simulink model "PV_MG_DroopMPPTV3_TwoFarms_VariableDT_VariableSampling"  (R2015a)
settings: Solver=ode3  StartTime=0.0  StopTime=inf  FixedStep=DT  RelTol=1e-3
undefined symbols (not defined in the file): CT, DT, Ion, Lithium
libraries: powerlib x61, powerlib_meascontrol x12, simulink x10, fuzblock x3, simulink_extras x3, re_lib x2, electricdrivelib x1
(part 2 of 2)

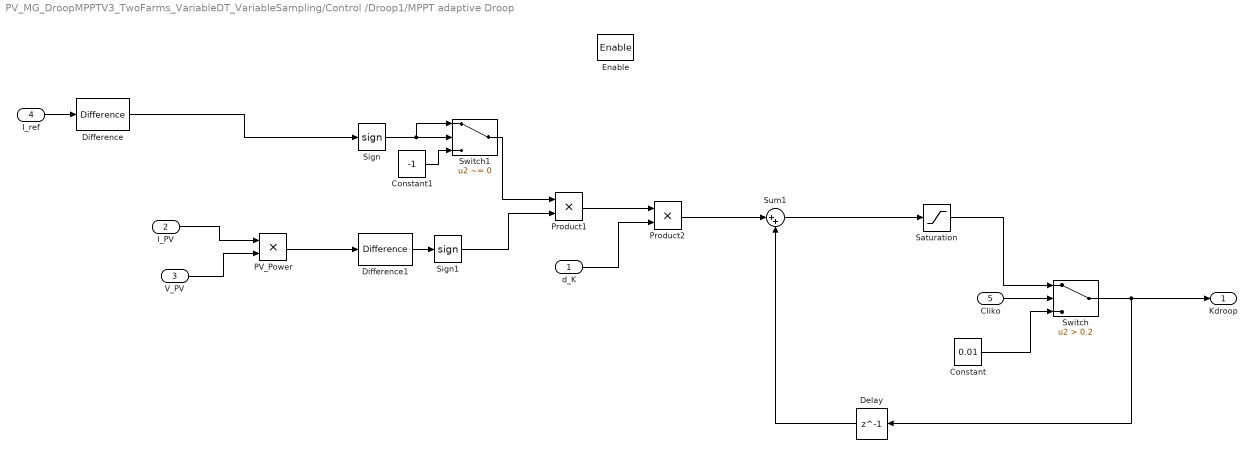
== system PV_MG_DroopMPPTV3_TwoFarms_VariableDT_VariableSampling/Control /Droop1/MPPT adaptive Droop ==
  d_K : Inport  SampleTime=CT
  I_PV : Inport  Port=2  SampleTime=CT
  V_PV : Inport  Port=3  SampleTime=CT
  I_ref : Inport  Port=4  SampleTime=CT
  "Cliko " : Inport  Port=5  SampleTime=CT
  Enable : EnablePort
  Constant : Constant  Value=0.01  SampleTime=CT
  Constant1 : Constant  Value=-1  SampleTime=CT
  Delay : Delay  DelayLength=1  InitialCondition=0  SampleTime=CT
  Difference : simulink/Discrete/Difference  ICPrevInput=0.0  InputProcessing=Inherited  OutMin=[]  OutMax=[]  OutDataType=fixdt(1, 16)  OutScaling=2^-10  DoSatur=off
  Difference1 : simulink/Discrete/Difference  ICPrevInput=0.0  InputProcessing=Inherited  OutMin=[]  OutMax=[]  OutDataType=fixdt(1, 16)  OutScaling=2^-10  DoSatur=off
  PV_Power : Product
  Product1 : Product
  Product2 : Product
  Saturation : Saturate  UpperLimit=4  LowerLimit=0
  Sign : Signum
  Sign1 : Signum
  Sum1 : Sum  Inputs=|++
  Switch : Switch  Criteria=u2 > Threshold  Threshold=0.2
  Switch1 : Switch  Criteria=u2 ~= 0  Threshold=0.1
  Kdroop : Outport  SampleTime=CT
  wires:
  I_ref/1 -> Difference/1
  V_PV/1 -> PV_Power/2
  I_PV/1 -> PV_Power/1
  Difference/1 -> Sign/1
  Switch1/1 -> Product1/1
  Constant1/1 -> Switch1/3
  Sign/1 -> Switch1/2, Switch1/1
  Saturation/1 -> Switch/1
  Constant/1 -> Switch/3
  Sum1/1 -> Saturation/1
  Delay/1 -> Sum1/2
  Product2/1 -> Sum1/1
  d_K/1 -> Product2/2
  Product1/1 -> Product2/1
  Sign1/1 -> Product1/2
  Difference1/1 -> Sign1/1
  PV_Power/1 -> Difference1/1
  Switch/1 -> Delay/1, Kdroop/1
  "Cliko "/1 -> Switch/2

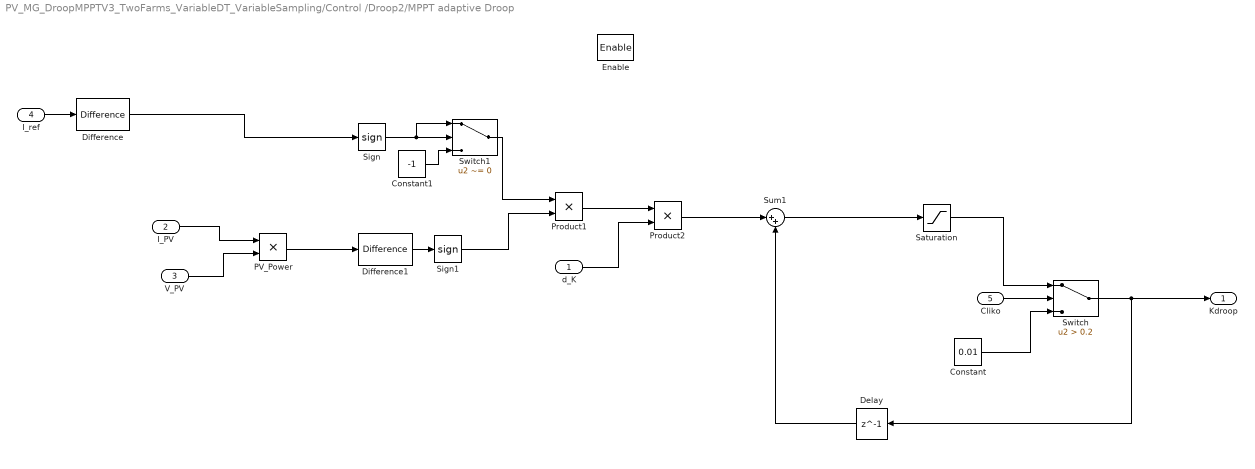
== system PV_MG_DroopMPPTV3_TwoFarms_VariableDT_VariableSampling/Control /Droop2/MPPT adaptive Droop ==
  d_K : Inport  SampleTime=CT
  I_PV : Inport  Port=2  SampleTime=CT
  V_PV : Inport  Port=3  SampleTime=CT
  I_ref : Inport  Port=4  SampleTime=CT
  "Cliko " : Inport  Port=5  SampleTime=CT
  Enable : EnablePort
  Constant : Constant  Value=0.01  SampleTime=CT
  Constant1 : Constant  Value=-1  SampleTime=CT
  Delay : Delay  DelayLength=1  InitialCondition=0  SampleTime=CT
  Difference : simulink/Discrete/Difference  ICPrevInput=0.0  InputProcessing=Inherited  OutMin=[]  OutMax=[]  OutDataType=fixdt(1, 16)  OutScaling=2^-10  DoSatur=off
  Difference1 : simulink/Discrete/Difference  ICPrevInput=0.0  InputProcessing=Inherited  OutMin=[]  OutMax=[]  OutDataType=fixdt(1, 16)  OutScaling=2^-10  DoSatur=off
  PV_Power : Product
  Product1 : Product
  Product2 : Product
  Saturation : Saturate  UpperLimit=4  LowerLimit=0
  Sign : Signum
  Sign1 : Signum
  Sum1 : Sum  Inputs=|++
  Switch : Switch  Criteria=u2 > Threshold  Threshold=0.2
  Switch1 : Switch  Criteria=u2 ~= 0  Threshold=0.1
  Kdroop : Outport  SampleTime=CT
  wires:
  I_ref/1 -> Difference/1
  V_PV/1 -> PV_Power/2
  I_PV/1 -> PV_Power/1
  Difference/1 -> Sign/1
  Switch1/1 -> Product1/1
  Constant1/1 -> Switch1/3
  Sign/1 -> Switch1/2, Switch1/1
  Saturation/1 -> Switch/1
  Constant/1 -> Switch/3
  Sum1/1 -> Saturation/1
  Delay/1 -> Sum1/2
  Product2/1 -> Sum1/1
  d_K/1 -> Product2/2
  Product1/1 -> Product2/1
  Sign1/1 -> Product1/2
  Difference1/1 -> Sign1/1
  PV_Power/1 -> Difference1/1
  Switch/1 -> Delay/1, Kdroop/1
  "Cliko "/1 -> Switch/2

== system PV_MG_DroopMPPTV3_TwoFarms_VariableDT_VariableSampling/Control /Battery Control/Bi-Current Controller/Fuzzy Control ==
  note: Filterout oscillations due to switching frequency
  I_ref : Inport
  I_measured : Inport  Port=2
  Action Port : ActionPort  ActionType=else
  Constant : Constant
  Constant1 : Constant  Value=0
  Discrete Filter1 : DiscreteFilter  Numerator=[1 -1]  Denominator=[1]
  First-Order Filter : powerlib_meascontrol/Filters/First-Order Filter  FilterType=Lowpass  Tc=1/8000  Ts=DT  Initialize=off  Vac_Init=[0, 0, 60]  Vdc_Init=0  PlotResponse=off  FreqRange="[0,  5000,  1]"
  Fuzzy Logic Controller : fuzblock/Fuzzy Logic  Controller  fis=ZIloop5
  Mux : Mux  Inputs=2
  PWM Generator (DC-DC) : powerlib_meascontrol/Pulse & Signal Generators/PWM Generator (DC-DC)  Fsw=10000  Ts=DT
  Saturation : Saturate  UpperLimit=0.8  LowerLimit=0
  Saturation1 : Saturate  UpperLimit=100  LowerLimit=-100
  Saturation2 : Saturate  UpperLimit=10  LowerLimit=-10
  Sum : Sum  Inputs=|+-
  Sum1 : Sum  Inputs=|++
  G : Outport
  lamp : Outport  Port=2  SourceOfInitialOutputValue=Input signal  InitialOutput=1
  D1 : Outport  Port=3
  wires:
  Mux/1 -> Fuzzy Logic Controller/1
  Fuzzy Logic Controller/1 -> Sum1/1
  I_ref/1 -> Sum/1
  Constant/1 -> lamp/1
  Saturation/1 -> D1/1, PWM Generator (DC-DC)/1
  PWM Generator (DC-DC)/1 -> G/1
  Sum/1 -> Saturation1/1
  Saturation1/1 -> Mux/1, Discrete Filter1/1
  Discrete Filter1/1 -> Saturation2/1
  Saturation2/1 -> Mux/2
  I_measured/1 -> First-Order Filter/1
  First-Order Filter/1 -> Sum/2
  Sum1/1 -> Saturation/1
  Constant1/1 -> Sum1/2

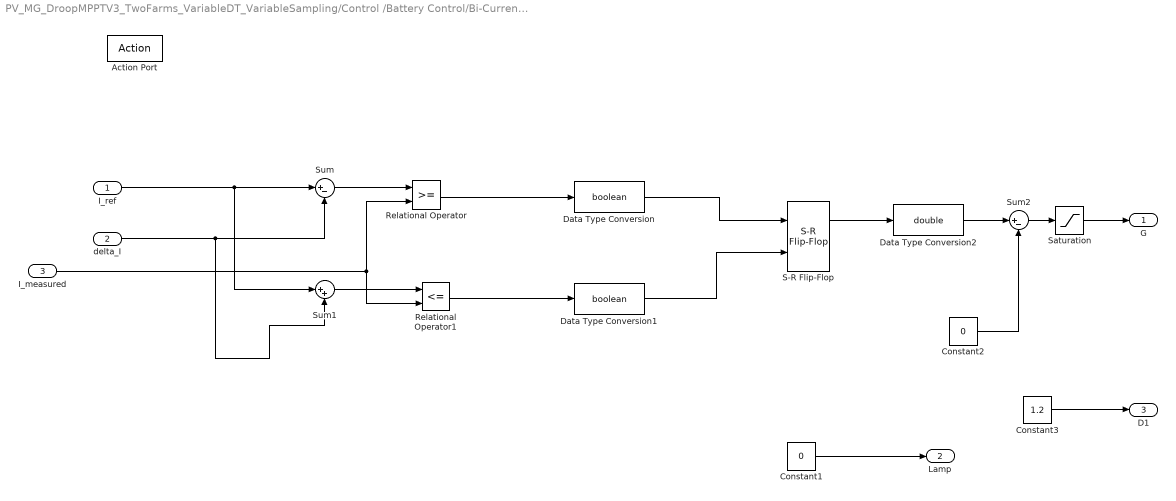
== system PV_MG_DroopMPPTV3_TwoFarms_VariableDT_VariableSampling/Control /Battery Control/Bi-Current Controller/Hysteric Control ==
  I_ref : Inport
  delta_I : Inport  Port=2
  I_measured : Inport  Port=3
  Action Port : ActionPort  ActionType=then
  Constant1 : Constant  Value=0
  Constant2 : Constant  Value=0
  Constant3 : Constant  Value=1.2
  Data Type Conversion : DataTypeConversion  OutDataTypeStr=boolean
  Data Type Conversion1 : DataTypeConversion  OutDataTypeStr=boolean
  Data Type Conversion2 : DataTypeConversion  OutDataTypeStr=double
  Relational Operator : RelationalOperator  OutDataTypeStr=boolean  ZeroCross=off
  Relational Operator1 : RelationalOperator  Operator=<=  OutDataTypeStr=boolean  ZeroCross=off
  S-R Flip-Flop : simulink_extras/Flip Flops/S-R Flip-Flop  initial_condition=0
  Saturation : Saturate  UpperLimit=1  LowerLimit=0
  Sum : Sum  Inputs=|+-
  Sum1 : Sum  Inputs=|++
  Sum2 : Sum  Inputs=|+-
  G : Outport
  Lamp : Outport  Port=2  InitialOutput=1
  D1 : Outport  Port=3
  wires:
  I_ref/1 -> Sum1/1, Sum/1
  delta_I/1 -> Sum/2, Sum1/2
  Data Type Conversion/1 -> S-R Flip-Flop/1
  Data Type Conversion1/1 -> S-R Flip-Flop/2
  Sum/1 -> Relational Operator/1
  Relational Operator/1 -> Data Type Conversion/1
  Relational Operator1/1 -> Data Type Conversion1/1
  Sum1/1 -> Relational Operator1/1
  I_measured/1 -> Relational Operator/2, Relational Operator1/2
  Constant1/1 -> Lamp/1
  Data Type Conversion2/1 -> Sum2/1
  Constant2/1 -> Sum2/2
  Sum2/1 -> Saturation/1
  Saturation/1 -> G/1
  Constant3/1 -> D1/1
  S-R Flip-Flop/1 -> Data Type Conversion2/1

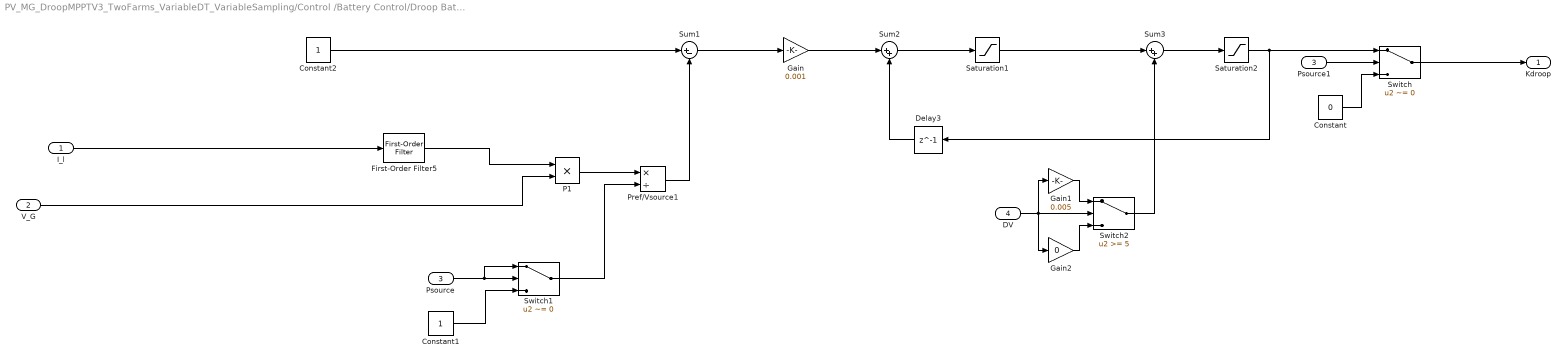
== system PV_MG_DroopMPPTV3_TwoFarms_VariableDT_VariableSampling/Control /Battery Control/Droop Batt/Enabled Subsystem ==
  I_l : Inport
  V_G : Inport  Port=2
  Psource : Inport  Port=3
  DV : Inport  Port=4
  Constant : Constant  Value=0  SampleTime=0
  Constant1 : Constant  SampleTime=0
  Constant2 : Constant  SampleTime=0
  Delay3 : Delay  DelayLength=1
  First-Order Filter5 : powerlib_meascontrol/Filters/First-Order Filter  FilterType=Lowpass  Tc=1/20000  Ts=DT  Initialize=off  Vac_Init=[0, 0, 60]  Vdc_Init=0  PlotResponse=off  FreqRange="[0,  5000,  1]"
  Gain : Gain  Gain=0.001
  Gain1 : Gain  Gain=0.005
  Gain2 : Gain  Gain=0
  P1 : Product
  Pref/Vsource1 : Product  Inputs=*/
  Psource1 : InportShadow  Port=3
  Saturation1 : Saturate  UpperLimit=10  LowerLimit=0
  Saturation2 : Saturate  UpperLimit=10  LowerLimit=0
  Sum1 : Sum  Inputs=|+-
  Sum2 : Sum  Inputs=|++
  Sum3 : Sum  Inputs=|++
  Switch : Switch  Criteria=u2 ~= 0
  Switch1 : Switch  Criteria=u2 ~= 0
  Switch2 : Switch  Threshold=5
  Kdroop : Outport
  wires:
  Delay3/1 -> Sum2/2
  Constant1/1 -> Switch1/3
  Switch1/1 -> Pref/Vsource1/2
  Psource/1 -> Switch1/2, Switch1/1
  Constant/1 -> Switch/3
  Psource1/1 -> Switch/2
  Switch/1 -> Kdroop/1
  Gain/1 -> Sum2/1
  Sum1/1 -> Gain/1
  Constant2/1 -> Sum1/1
  First-Order Filter5/1 -> P1/1
  I_l/1 -> First-Order Filter5/1
  Sum2/1 -> Saturation1/1
  Pref/Vsource1/1 -> Sum1/2
  P1/1 -> Pref/Vsource1/1
  V_G/1 -> P1/2
  DV/1 -> Gain2/1, Gain1/1, Switch2/2
  Gain1/1 -> Switch2/1
  Gain2/1 -> Switch2/3
  Saturation1/1 -> Sum3/1
  Sum3/1 -> Saturation2/1
  Switch2/1 -> Sum3/2
  Saturation2/1 -> Delay3/1, Switch/1
